simulink model "segway_planar_linmod"  (R2023a)
settings: Solver=VariableStepAuto  StartTime=0.0  StopTime=10.0  RelTol=1e-3
values from neighbouring files (symbols this model uses):
  Cr2w = Cw2r^-1    [segway_ini.m]    (also in segway_planar_ini.m)
  Cw2r = [p.r/2     p.r/2;          p.r/p.b, -p.r/p.b]    [segway_ini.m]    (also in segway_planar_ini.m = [p.r])
  p = get_segway_params()    [segway_ini.m]    (also in segway_planar_ini.m)
  s = 2*pi    (= 6.28318530718)    [segway_planar_ini.m]
libraries: cstblocks x1
settings Model: Creator=Michael Peter  LastModifiedBy=Michael Peter

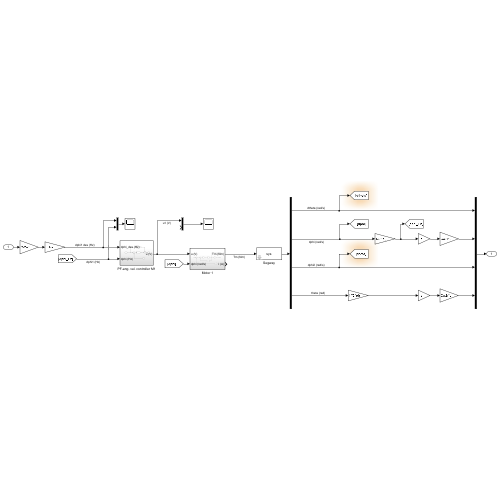
[thumbnail: Simulink's stored preview of the top-level diagram]
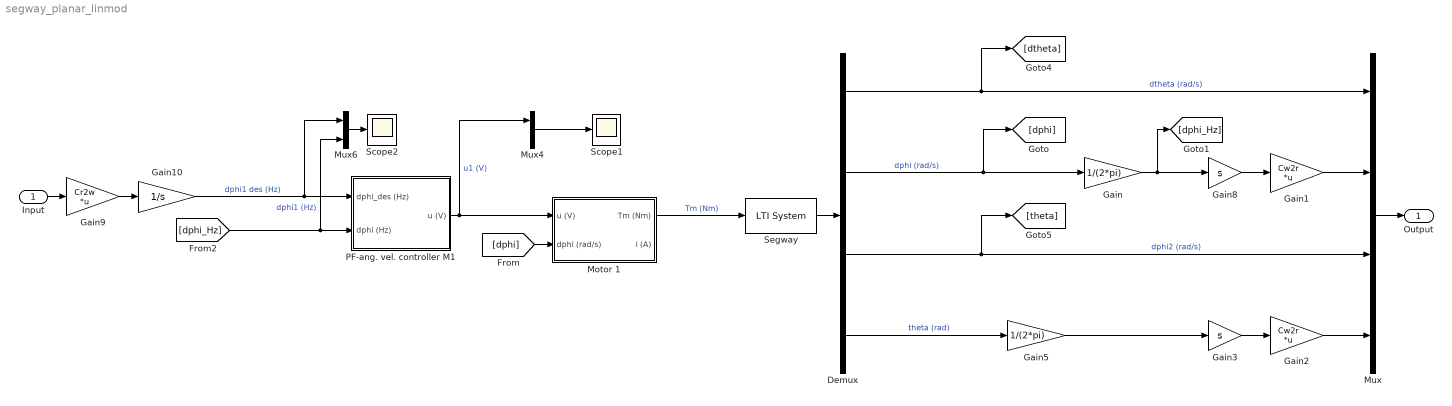
== system segway_planar_linmod ==
  Input : Inport
  Demux : Demux
  Gain : Gain  Gain=1/(2*pi)
  Gain1 : Gain  Gain=Cw2r  Multiplication=Matrix(K*u)
  Gain10 : Gain  Gain=1/s
  Gain2 : Gain  Gain=Cw2r  Multiplication=Matrix(K*u)
  Gain3 : Gain  Gain=s
  Gain5 : Gain  Gain=1/(2*pi)
  Gain8 : Gain  Gain=s
  Gain9 : Gain  Gain=Cr2w  Multiplication=Matrix(K*u)
  Motor 1 : Subsystem
  Mux : Mux
  Mux4 : Mux  Inputs=2
  Mux6 : Mux  Inputs=2
  PF-ang. vel. controller M1 : Subsystem
  Scope1 : Scope
  Scope2 : Scope
  Segway : cstblocks/LTI System  sys=sys  IC=x0
  Output : Outport
  wires:
  Gain10/1 -> PF-ang. vel. controller M1/1(dphi_des (Hz)), Mux6/1  "dphi1 des (Hz)"
  Gain8/1 -> Gain1/1
  Gain5/1 -> Gain3/1
  Input/1 -> Gain9/1
  Gain9/1 -> Gain10/1
  Mux/1 -> Output/1
  Motor 1/1(Tm (Nm)) -> Segway/1  "Tm (Nm)"
  Demux/3 -> [theta], Mux/3  "dphi2 (rad/s)"
  [dphi] -> Motor 1/2(dphi (rad/s))
  Demux/4 -> Gain5/1  "theta (rad)"
  Mux6/1 -> Scope2/1
  [dphi_Hz] -> PF-ang. vel. controller M1/2(dphi (Hz)), Mux6/2  "dphi1 (Hz)"
  Gain/1 -> Gain8/1, [dphi_Hz]
  Mux4/1 -> Scope1/1
  Demux/1 -> [dtheta], Mux/1  "dtheta (rad/s)"
  Gain3/1 -> Gain2/1
  Segway/1 -> Demux/1
  PF-ang. vel. controller M1/1(u (V)) -> Motor 1/1(u (V)), Mux4/1  "u1 (V)"
  Demux/2 -> [dphi], Gain/1  "dphi (rad/s)"
  Gain1/1 -> Mux/2
  Gain2/1 -> Mux/4

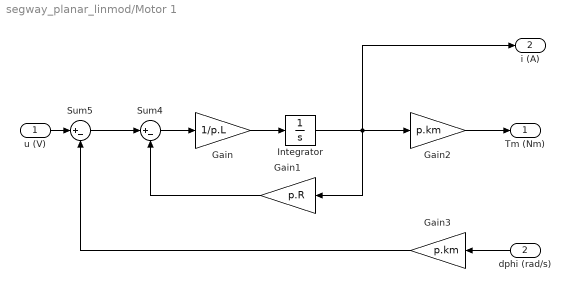
== system segway_planar_linmod/Motor 1 ==
  u (V) : Inport
  dphi (rad/s) : Inport  Port=2
  Gain : Gain  Gain=1/p.L
  Gain1 : Gain  Gain=p.R
  Gain2 : Gain  Gain=p.km
  Gain3 : Gain  Gain=p.km
  Integrator : Integrator
  Sum4 : Sum  Inputs=|+-
  Sum5 : Sum  Inputs=|+-
  Tm (Nm) : Outport
  i (A) : Outport  Port=2
  wires:
  Integrator/1 -> Gain1/1, i (A)/1, Gain2/1
  Gain1/1 -> Sum4/2
  Gain3/1 -> Sum5/2
  u (V)/1 -> Sum5/1
  Sum5/1 -> Sum4/1
  Sum4/1 -> Gain/1
  Gain/1 -> Integrator/1
  dphi (rad/s)/1 -> Gain3/1
  Gain2/1 -> Tm (Nm)/1

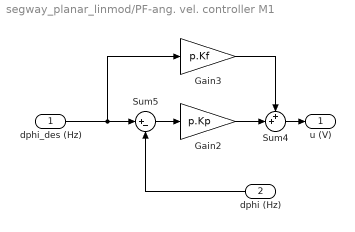
== system segway_planar_linmod/PF-ang. vel. controller M1 ==
  dphi_des (Hz) : Inport
  dphi (Hz) : Inport  Port=2
  Gain2 : Gain  Gain=p.Kp
  Gain3 : Gain  Gain=p.Kf
  Sum4 : Sum  Inputs=++|
  Sum5 : Sum  Inputs=|+-
  u (V) : Outport
  wires:
  Sum5/1 -> Gain2/1
  dphi_des (Hz)/1 -> Gain3/1, Sum5/1
  dphi (Hz)/1 -> Sum5/2
  Gain3/1 -> Sum4/1
  Gain2/1 -> Sum4/2
  Sum4/1 -> u (V)/1
